simulink model "PMS_Motor_level4eZDSPF2812"  (Simulink 6.5)
settings: Solver=FixedStepDiscrete  StartTime=0.0  StopTime=0.3  RelTol=1e-3
libraries: simulink x13, tiiqmathlib x9, c28xdmclib x8, c281xdspchiplib x5, memblks x4, c2000tgtpreflib x1
CloseFcn:
  | rtwprivate ssgencode ModelCloseRequest Simple_DC_Motor
settings Model: Creator=JacobF  LastModifiedBy=JacobF  ProdHWDeviceType=TI C2000
settings DataIOCC: SaveOutput=off  SaveTime=off  SignalLoggingName=DataLog
settings OptimizationCC: OptimizeModelRefInitCode=on  LifeSpan=1
settings DebuggingCC: ReadBeforeWriteMsg=DisableAll  MultiTaskDSMMsg=warning  MultiTaskCondExecSysMsg=none  ParameterPrecisionLossMsg=none  StrictBusMsg=ErrorLevel1
settings HardwareCC: ProdBitPerChar=16  ProdBitPerInt=16  ProdIntDivRoundTo=Zero  ProdEndianess=LittleEndian  ProdWordSize=16  ProdHWDeviceType=TI C2000  TargetHWDeviceType=32-bit Generic
settings RTWCC: SystemTargetFile=ti_c2000_ert.tlc  GenCodeOnly=on  TemplateMakefile=ti_c2000_ert.tmf  Description=Embedded Target for TI C2000 DSP (ERT)  GenerateReport=on  ProcessScript=ti_c2000_ert_make_rtw_hook  IncludeHyperlinkInReport=on  LaunchReport=on
settings CodeAppCC: IgnoreCustomStorageClasses=off
settings STFCustomTargetCC: TargetFcnLib=ansi_tfl_tmw.mat  GenFloatMathFcnCalls=ANSI_C  ModelReferenceCompliant=off  CombineOutputUpdateFcns=on  ERTCustomFileBanners=on  SystemTargetFile=ti_c2000_ert.tlc
settings ERTTargetCC: TargetFcnLib=ansi_tfl_tmw.mat  GenFloatMathFcnCalls=ANSI_C  ModelReferenceCompliant=off  SupportContinuousTime=on  SupportNonInlinedSFcns=on  InlinedParameterPlacement=NonHierarchical  ERTCustomFileTemplate=example_file_process.tlc

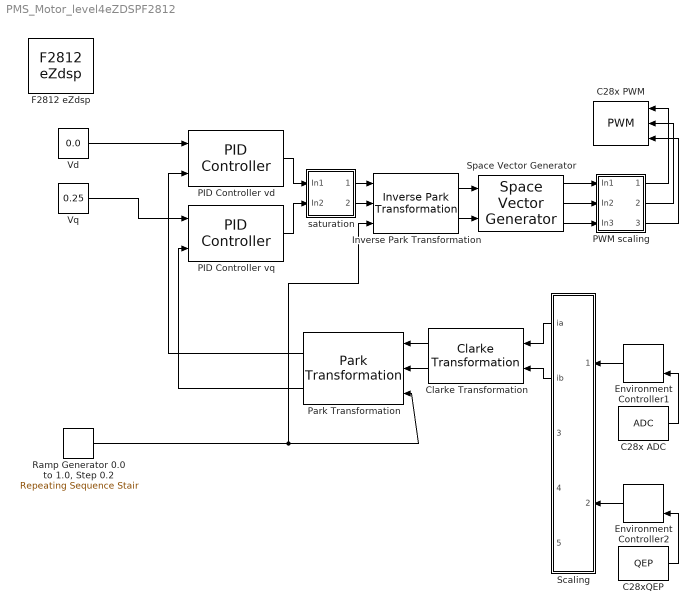
== system PMS_Motor_level4eZDSPF2812 ==
  C28x ADC : c281xdspchiplib/ADC  useModule=A  useMode=Sequential  sourceSOC=Software  Ts=-1  dType=uint16  postInterrupt=off  numConversionsSingle=3  numConversionsDouble=1  conv0=ADCINB0  conv1=ADCINB1  conv2=ADCINB2  conv3=ADCINB3  conv4=ADCINA4  conv5=ADCINA5  conv6=ADCINB6  conv7=ADCINA7  conv8=ADCINB0  conv9=ADCINB1  conv10=ADCINB2  conv11=ADCINB3  conv12=ADCINB4  conv13=ADCINB5  conv14=ADCINB6  conv15=ADCINB7  convAB0=ADCINA0 and ADCINB0  convAB1=ADCINA1 and ADCINB1  convAB2=ADCINA5 and ADCINB5  convAB3=ADCINA1 and ADCINB1  convAB4=ADCINA1 and ADCINB1  convAB5=ADCINA1 and ADCINB1  convAB6=ADCINA1 and ADCINB1  convAB7=ADCINA1 and ADCINB1  convA0=ADCINA0  convA1=ADCINA1  convA2=ADCINA7  convA3=ADCINA3  convA4=ADCINA4  convA5=ADCINA5  convA6=ADCINA6  convA7=ADCINA7  convB0=ADCINB0  convB1=ADCINB1  convB2=ADCINB2  convB3=ADCINB3  convB4=ADCINB4  convB5=ADCINB5  convB6=ADCINB6  convB7=ADCINB7  c28xmultiPort=off
  C28x PWM : c281xdspchiplib/PWM  Orientation=left  useModule=A  timerSource=Specify via dialog  timerPeriod=(2^12)+1  waveformType=Symmetric  periodUnits=Clock cycles  unit1Status=on  unit1Source=Input port  unit1Value=4096  unit2Status=on  unit2Source=Input port  unit2Value=4096  unit3Status=on  unit3Source=Input port  unit3Value=4096  dutyCycleUnits=Clock cycles  logicSource=Specify via dialog  unit1_1Logic=Active high  unit1_2Logic=Active low  unit2_1Logic=Active high  unit2_2Logic=Active low  unit3_1Logic=Active high  unit3_2Logic=Active low  enableDeadband1=on  enableDeadband2=on  enableDeadband3=on  deadbandPrescaler=8  deadbandPeriodSource=Specify via dialog  deadbandPeriod=15  adcstartEvent=None
  C28xQEP : c281xdspchiplib/QEP  useModule=A  countingMode=Counter  positiveRotation=Clockwise  initialCount=0  encoderResolution=1024  sampleTime=5e-5  dataType=uint16
  Clarke Transformation : c28xdmclib/Clarke Transformation  Orientation=left
  Environment Controller1 : simulink/Signal Routing/Environment Controller  Orientation=left  SystemSampleTime=-1
  Environment Controller2 : simulink/Signal Routing/Environment Controller  Orientation=left  SystemSampleTime=-1
  F2812 eZdsp : c2000tgtpreflib/F2812 eZdsp  Tag=C2000 TARGET PREFERENCES BLOCK  SystemSampleTime=-1
  Inverse Park Transformation : c28xdmclib/Inverse Park Transformation
  PID Controller vd : c28xdmclib/PID Controller  proportionalGain=0.2  integralGain=0.002  correctionGain=0.002  derivativeGain=0  minOutput=-1  maxOutput=1
  PID Controller vq : c28xdmclib/PID Controller  proportionalGain=0.2  integralGain=0.002  correctionGain=0.002  derivativeGain=0  minOutput=-1  maxOutput=1
  PWM scaling : Subsystem
  Park Transformation : c28xdmclib/Park Transformation  Orientation=left
  "Ramp Generator 0.0 to 1.0, Step 0.2" : simulink/Sources/Repeating Sequence Stair  SystemSampleTime=-1  OutValues=[0.0:0.0005:1.0]  tsamp=0.00005  OutputDataTypeScalingMode=Specify via dialog  OutDataType=sfix(32)  ConRadixGroup=Use Specified Scaling  OutScaling=2^-17
  Scaling : Subsystem  Orientation=left
  Space Vector Generator : c28xdmclib/Space Vector Generator
  Vd : Constant  Value=0.0  OutDataTypeMode=Specify via dialog  OutDataType=sfix(32)  ConRadixGroup=Use specified scaling  OutScaling=2^-17  SampleTime=inf  FramePeriod=inf
  Vq : Constant  Value=0.25  OutDataTypeMode=Specify via dialog  OutDataType=sfix(32)  ConRadixGroup=Use specified scaling  OutScaling=2^-17  SampleTime=inf  FramePeriod=inf
  saturation : Subsystem
  wires:
  Inverse Park Transformation/1 -> Space Vector Generator/1
  Inverse Park Transformation/2 -> Space Vector Generator/2
  Space Vector Generator/1 -> PWM scaling/1(In1)
  Space Vector Generator/2 -> PWM scaling/2(In2)
  Space Vector Generator/3 -> PWM scaling/3(In3)
  PWM scaling/1(Out1) -> C28x PWM/1
  PWM scaling/2(Out2) -> C28x PWM/2
  PWM scaling/3(Out3) -> C28x PWM/3
  C28xQEP/1 -> Environment Controller2/2
  Environment Controller1/1 -> Scaling/1(ADC)
  C28x ADC/1 -> Environment Controller1/2
  Environment Controller2/1 -> Scaling/2(QEP)
  Scaling/1(ia) -> Clarke Transformation/1
  Scaling/2(ib) -> Clarke Transformation/2
  Clarke Transformation/1 -> Park Transformation/1
  Clarke Transformation/2 -> Park Transformation/2
  PID Controller vd/1 -> saturation/1(In1)
  PID Controller vq/1 -> saturation/2(In2)
  Vd/1 -> PID Controller vd/1
  Park Transformation/1 -> PID Controller vd/2
  Park Transformation/2 -> PID Controller vq/2
  saturation/1(Out1) -> Inverse Park Transformation/1
  saturation/2(Out2) -> Inverse Park Transformation/2
  Vq/1 -> PID Controller vq/1
  "Ramp Generator 0.0 to 1.0, Step 0.2"/1 -> Inverse Park Transformation/3, Park Transformation/3

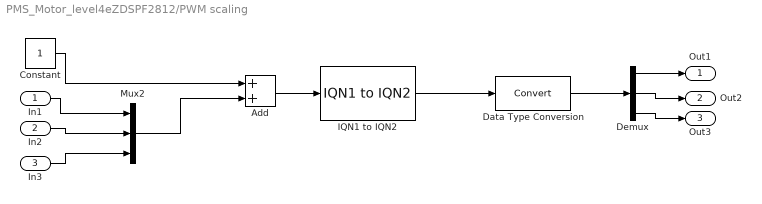
== system PMS_Motor_level4eZDSPF2812/PWM scaling ==
  In1 : Inport
  In2 : Inport  Port=2
  In3 : Inport  Port=3
  Add : Sum  OutScaling=2^-10
  Constant : Constant  Value=1  OutDataTypeMode=Specify via dialog  OutDataType=sfix(32)  ConRadixGroup=Use specified scaling  OutScaling=2^-17  SampleTime=inf  FramePeriod=inf
  Data Type Conversion : DataTypeConversion  OutDataTypeMode=uint16  ConvertRealWorld=Stored Integer (SI)
  Demux : Demux  Outputs=3
  IQN1 to IQN2 : tiiqmathlib/IQN1 to IQN2  New_Q=11
  Mux2 : Mux  Inputs=3
  Out1 : Outport
  Out2 : Outport  Port=2
  Out3 : Outport  Port=3
  wires:
  In1/1 -> Mux2/1
  Add/1 -> IQN1 to IQN2/1
  Constant/1 -> Add/1
  IQN1 to IQN2/1 -> Data Type Conversion/1
  In3/1 -> Mux2/3
  In2/1 -> Mux2/2
  Mux2/1 -> Add/2
  Data Type Conversion/1 -> Demux/1
  Demux/3 -> Out3/1
  Demux/2 -> Out2/1
  Demux/1 -> Out1/1

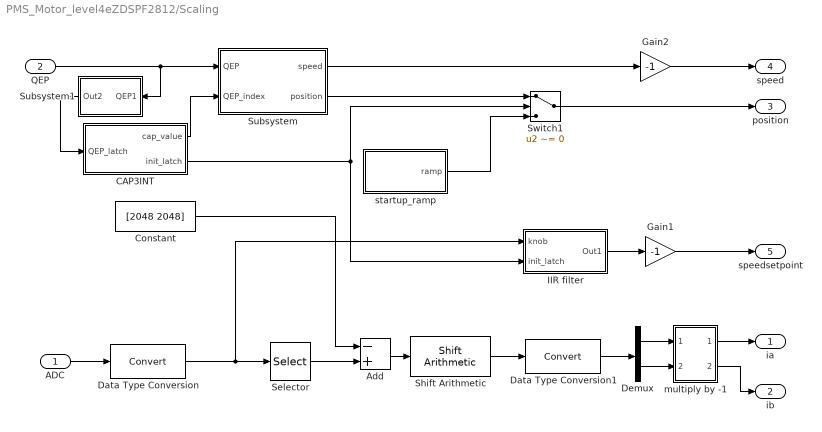
== system PMS_Motor_level4eZDSPF2812/Scaling ==
  ADC : Inport
  QEP : Inport  Port=2
  Add : Sum  Inputs=-+  OutScaling=2^-10
  CAP3INT : Subsystem
  Constant : Constant  Value=[2048 2048]  OutDataTypeMode=int32  OutDataType=sfix(32)  ConRadixGroup=Use specified scaling  OutScaling=2^-12  SampleTime=inf  FramePeriod=inf
  Data Type Conversion : DataTypeConversion  OutDataTypeMode=int32  OutDataType=sfix(32)  OutScaling=2^-12  ConvertRealWorld=Stored Integer (SI)
  Data Type Conversion1 : DataTypeConversion  OutDataTypeMode=Specify via dialog  OutDataType=sfix(32)  OutScaling=2^-17  ConvertRealWorld=Stored Integer (SI)
  Demux : Demux  Outputs=2
  Gain1 : Gain  Gain=-1
  Gain2 : Gain  Gain=-1
  IIR filter : Subsystem
  Selector : Selector  InputType=Vector  ElementSrc=Internal  Elements=[1 2]  RowSrc=Internal  Rows=1  ColumnSrc=Internal  Columns=1  InputPortWidth=3  IndexIsStartValue=off
  Shift Arithmetic : simulink/Logic and Bit Operations/Shift Arithmetic  SystemSampleTime=-1  nBitShiftRight=-6  nBinPtShiftRight=0
  Subsystem : Subsystem
  Subsystem1 : Subsystem  Orientation=left
      settings: RTWMemSecFuncInitTerm=Default  RTWMemSecFuncExecute=Default  RTWMemSecDataConstants=Default  RTWMemSecDataInternal=Default  RTWMemSecDataParameters=Default
  Switch1 : Switch  Criteria=u2 ~= 0
  multiply by -1 : Subsystem
  startup_ramp : Subsystem
  ia : Outport
  ib : Outport  Port=2
  position : Outport  Port=3
  speed : Outport  Port=4
  speedsetpoint : Outport  Port=5
  wires:
  Subsystem1/1(Out2) -> CAP3INT/1(QEP_latch)
  Switch1/1 -> position/1
  ADC/1 -> Data Type Conversion/1
  QEP/1 -> Subsystem/1(QEP), Subsystem1/1(QEP1)
  multiply by -1/2(Out2) -> ib/1
  multiply by -1/1(Out1) -> ia/1
  Demux/2 -> multiply by -1/2(In2)
  Demux/1 -> multiply by -1/1(In1)
  Data Type Conversion1/1 -> Demux/1
  Shift Arithmetic/1 -> Data Type Conversion1/1
  Add/1 -> Shift Arithmetic/1
  Selector/1 -> Add/2
  Constant/1 -> Add/1
  IIR filter/1(Out1) -> Gain1/1
  Data Type Conversion/1 -> IIR filter/1(knob), Selector/1
  Subsystem/2(position) -> Switch1/1
  Subsystem/1(speed) -> Gain2/1
  startup_ramp/1(ramp) -> Switch1/3
  CAP3INT/2(init_latch) -> IIR filter/2(init_latch), Switch1/2
  CAP3INT/1(cap_value) -> Subsystem/2(QEP_index)
  Gain2/1 -> speed/1
  Gain1/1 -> speedsetpoint/1

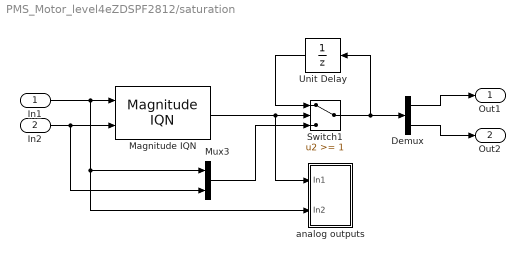
== system PMS_Motor_level4eZDSPF2812/saturation ==
  In1 : Inport
  In2 : Inport  Port=2
  Demux : Demux  Outputs=2
  Magnitude IQN : tiiqmathlib/Magnitude IQN
  Mux3 : Mux  Inputs=2
  Switch1 : Switch  Threshold=1
  Unit Delay : UnitDelay  Orientation=left  X0=[0 0]  SampleTime=-1
  analog outputs : Subsystem
  Out1 : Outport
  Out2 : Outport  Port=2
  wires:
  Magnitude IQN/1 -> Switch1/2, analog outputs/1(In1)
  In1/1 -> Magnitude IQN/1, Mux3/1, analog outputs/2(In2)
  In2/1 -> Magnitude IQN/2, Mux3/2
  Mux3/1 -> Switch1/3
  Switch1/1 -> Unit Delay/1, Demux/1
  Unit Delay/1 -> Switch1/1
  Demux/1 -> Out1/1
  Demux/2 -> Out2/1

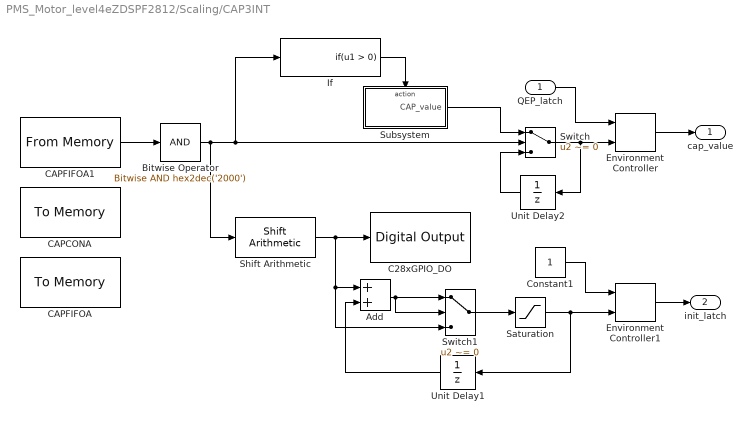
== system PMS_Motor_level4eZDSPF2812/Scaling/CAP3INT ==
  QEP_latch : Inport
  Add : Sum  OutDataTypeMode=uint16  OutScaling=2^-10
  Bitwise Operator : simulink/Logic and Bit Operations/Bitwise Operator  logicop=AND  UseBitMask=on  BitMask=hex2dec('2000')  BitMaskRealWorld=Stored Integer
  C28xGPIO_DO : c281xdspchiplib/Digital Output  useIOPort=GPIOB  GPIO_Bit0=off  GPIO_Bit1=off  GPIO_Bit2=off  GPIO_Bit3=off  GPIO_Bit4=off  GPIO_Bit5=off  GPIO_Bit6=off  GPIO_Bit7=off  GPIO_Bit8=off  GPIO_Bit9=on  GPIO_Bit10=off  GPIO_Bit11=off  GPIO_Bit12=off  GPIO_Bit13=off  GPIO_Bit14=off  GPIO_Bit15=off
  CAPCONA : memblks/To Memory  memAddressMask=7420  dType=uint16  useInitValue=on  initValue=hex2dec('1004')  useTermValue=off  termValue=0  isRealtimeEnabled=off  emitCCBeforeWrite=off  emitCCAfterWrite=off
  CAPFIFOA : memblks/To Memory  memAddressMask=7422  dType=uint16  useInitValue=on  initValue=hex2dec('1000')  useTermValue=off  termValue=0  isRealtimeEnabled=off  emitCCBeforeWrite=off  emitCCAfterWrite=off
  CAPFIFOA1 : memblks/From Memory  memAddressMask=7422  dType=uint16  Ts=-1  frameSize=1
  Constant1 : Constant  Value=1  OutDataTypeMode=uint16  OutDataType=sfix(16)  ConRadixGroup=Use specified scaling  OutScaling=2^0  SampleTime=inf  FramePeriod=inf
  Environment Controller : simulink/Signal Routing/Environment Controller  SystemSampleTime=-1
  Environment Controller1 : simulink/Signal Routing/Environment Controller  SystemSampleTime=-1
  If : If  ShowElse=off
  Saturation : Saturate  UpperLimit=1  LowerLimit=0
  Shift Arithmetic : simulink/Logic and Bit Operations/Shift Arithmetic  SystemSampleTime=-1  nBitShiftRight=13  nBinPtShiftRight=0
  Subsystem : Subsystem  TreatAsAtomicUnit=on
  Switch : Switch  Criteria=u2 ~= 0
  Switch1 : Switch  Criteria=u2 ~= 0  InputSameDT=on
  Unit Delay1 : UnitDelay  Orientation=left  SampleTime=-1
  Unit Delay2 : UnitDelay  Orientation=left  SampleTime=-1
  cap_value : Outport
  init_latch : Outport  Port=2
  wires:
  Constant1/1 -> Environment Controller1/1
  Environment Controller1/1 -> init_latch/1
  QEP_latch/1 -> Environment Controller/1
  Environment Controller/1 -> cap_value/1
  Saturation/1 -> Environment Controller1/2, Unit Delay1/1
  Switch1/1 -> Saturation/1
  Add/1 -> Switch1/1, Switch1/2
  Unit Delay1/1 -> Add/2
  Shift Arithmetic/1 -> Switch1/3, Add/1, C28xGPIO_DO/1
  Bitwise Operator/1 -> Shift Arithmetic/1, Switch/2, If/1
  If/1 -> Subsystem/Action
  Unit Delay2/1 -> Switch/3
  Switch/1 -> Environment Controller/2, Unit Delay2/1
  Subsystem/1(CAP_value) -> Switch/1
  CAPFIFOA1/1 -> Bitwise Operator/1

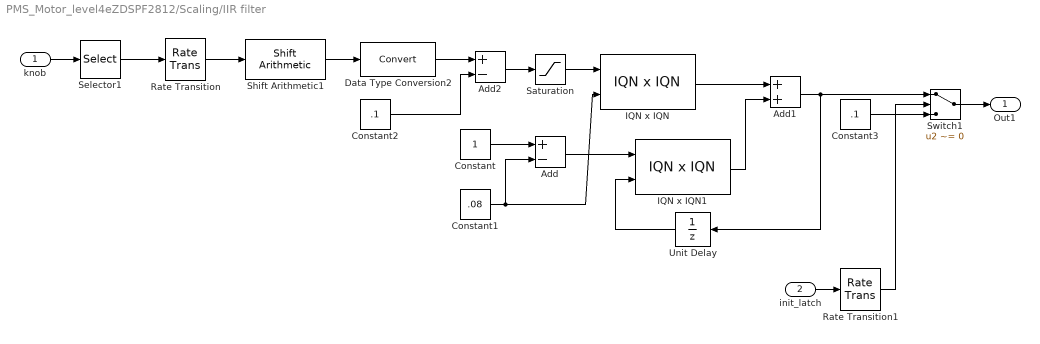
== system PMS_Motor_level4eZDSPF2812/Scaling/IIR filter ==
  knob : Inport
  init_latch : Inport  Port=2
  Add : Sum  Inputs=+-  OutScaling=2^-10
  Add1 : Sum  OutScaling=2^-10
  Add2 : Sum  Inputs=+-  OutScaling=2^-10
  Constant : Constant  Value=1  OutDataTypeMode=Specify via dialog  OutDataType=sfix(32)  ConRadixGroup=Use specified scaling  OutScaling=2^-17  SampleTime=inf  FramePeriod=inf
  Constant1 : Constant  Value=.08  OutDataTypeMode=Specify via dialog  OutDataType=sfix(32)  ConRadixGroup=Use specified scaling  OutScaling=2^-17  SampleTime=inf  FramePeriod=inf
  Constant2 : Constant  Value=.1  OutDataTypeMode=Specify via dialog  OutDataType=sfix(32)  ConRadixGroup=Use specified scaling  OutScaling=2^-17  SampleTime=inf  FramePeriod=inf
  Constant3 : Constant  Value=.1  OutDataTypeMode=Specify via dialog  OutDataType=sfix(32)  ConRadixGroup=Use specified scaling  OutScaling=2^-17  SampleTime=inf  FramePeriod=inf
  Data Type Conversion2 : DataTypeConversion  OutDataTypeMode=Specify via dialog  OutDataType=sfix(32)  OutScaling=2^-17  ConvertRealWorld=Stored Integer (SI)
  IQN x IQN : tiiqmathlib/IQN x IQN  multiplyOption=Multiply
  IQN x IQN1 : tiiqmathlib/IQN x IQN  multiplyOption=Multiply
  Rate Transition : RateTransition  Integrity=off  OutPortSampleTime=0.01
  Rate Transition1 : RateTransition  Integrity=off  OutPortSampleTime=0.01
  Saturation : Saturate  UpperLimit=1  LowerLimit=0
  Selector1 : Selector  InputType=Vector  ElementSrc=Internal  Elements=[3]  RowSrc=Internal  Rows=1  ColumnSrc=Internal  Columns=1  InputPortWidth=3  IndexIsStartValue=off
  Shift Arithmetic1 : simulink/Logic and Bit Operations/Shift Arithmetic  SystemSampleTime=-1  nBitShiftRight=-5  nBinPtShiftRight=0
  Switch1 : Switch  Criteria=u2 ~= 0
  Unit Delay : UnitDelay  Orientation=left  SampleTime=-1
  Out1 : Outport
  wires:
  Saturation/1 -> IQN x IQN/1
  Rate Transition/1 -> Shift Arithmetic1/1
  Rate Transition1/1 -> Switch1/2
  Switch1/1 -> Out1/1
  Constant3/1 -> Switch1/3
  init_latch/1 -> Rate Transition1/1
  Add2/1 -> Saturation/1
  Data Type Conversion2/1 -> Add2/1
  Constant2/1 -> Add2/2
  Shift Arithmetic1/1 -> Data Type Conversion2/1
  IQN x IQN1/1 -> Add1/2
  Unit Delay/1 -> IQN x IQN1/2
  Add1/1 -> Switch1/1, Unit Delay/1
  Add/1 -> IQN x IQN1/1
  IQN x IQN/1 -> Add1/1
  Constant1/1 -> IQN x IQN/2, Add/2
  Constant/1 -> Add/1
  knob/1 -> Selector1/1
  Selector1/1 -> Rate Transition/1

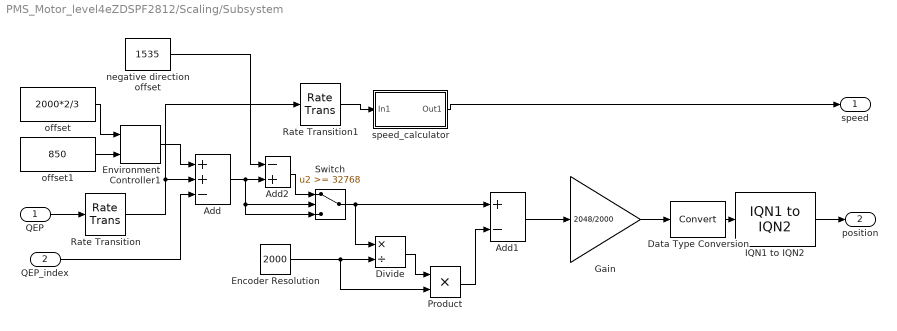
== system PMS_Motor_level4eZDSPF2812/Scaling/Subsystem ==
  QEP : Inport
  QEP_index : Inport  Port=2
  Add : Sum  Inputs=++-  OutScaling=2^-10
  Add1 : Sum  Inputs=+-  OutDataTypeMode=uint16  OutScaling=2^-10  RndMeth=Nearest
  Add2 : Sum  Inputs=-+  OutScaling=2^-10
  Data Type Conversion : DataTypeConversion  OutDataTypeMode=Specify via dialog  OutDataType=sfix(32)  OutScaling=2^-11  ConvertRealWorld=Stored Integer (SI)
  Divide : Product  Inputs=*/  OutDataTypeMode=uint16  OutScaling=2^-10
  Encoder Resolution : Constant  Value=2000  OutDataTypeMode=uint16  OutDataType=sfix(16)  ConRadixGroup=Use specified scaling  OutScaling=2^0  SampleTime=inf  FramePeriod=inf
  Environment Controller1 : simulink/Signal Routing/Environment Controller  SystemSampleTime=-1
  Gain : Gain  Gain=2048/2000  ParameterDataTypeMode=Specify via dialog  ParameterDataType=float('single')
  IQN1 to IQN2 : tiiqmathlib/IQN1 to IQN2  New_Q=17
  Product : Product  OutDataTypeMode=uint16  RndMeth=Zero
  Rate Transition : RateTransition
  Rate Transition1 : RateTransition
  Switch : Switch  Threshold=32768
  negative direction offset : Constant  Value=1535  OutDataTypeMode=uint16  OutDataType=sfix(16)  ConRadixGroup=Use specified scaling  OutScaling=2^0  SampleTime=inf  FramePeriod=inf
  offset : Constant  Value=2000*2/3  OutDataTypeMode=uint16  OutDataType=sfix(16)  ConRadixGroup=Use specified scaling  OutScaling=2^0  SampleTime=inf  FramePeriod=inf
  offset1 : Constant  Value=850  OutDataTypeMode=uint16  OutDataType=sfix(16)  ConRadixGroup=Use specified scaling  OutScaling=2^0  SampleTime=inf  FramePeriod=inf
  speed_calculator : Subsystem
  speed : Outport
  position : Outport  Port=2
  wires:
  offset1/1 -> Environment Controller1/2
  Environment Controller1/1 -> Add/1
  offset/1 -> Environment Controller1/1
  Add1/1 -> Gain/1
  Rate Transition1/1 -> speed_calculator/1(In1)
  Rate Transition/1 -> Add/2, Rate Transition1/1
  QEP_index/1 -> Add/3
  QEP/1 -> Rate Transition/1
  speed_calculator/1(Out1) -> speed/1
  Switch/1 -> Add1/1, Divide/1
  Add2/1 -> Switch/1
  negative direction offset/1 -> Add2/1
  IQN1 to IQN2/1 -> position/1
  Data Type Conversion/1 -> IQN1 to IQN2/1
  Gain/1 -> Data Type Conversion/1
  Product/1 -> Add1/2
  Divide/1 -> Product/1
  Encoder Resolution/1 -> Divide/2, Product/2
  Add/1 -> Add2/2, Switch/2, Switch/3

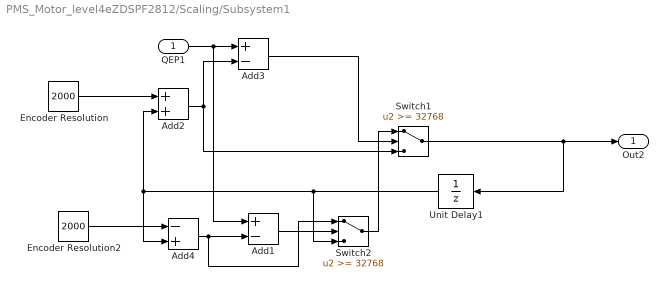
== system PMS_Motor_level4eZDSPF2812/Scaling/Subsystem1 ==
  QEP1 : Inport
  Add1 : Sum  Inputs=+-  OutDataTypeMode=uint16  OutScaling=2^-10
  Add2 : Sum  OutDataTypeMode=uint16  OutScaling=2^-10
  Add3 : Sum  Inputs=+-  OutDataTypeMode=uint16  OutScaling=2^-10
  Add4 : Sum  Inputs=-+  OutDataTypeMode=uint16  OutScaling=2^-10
  Encoder Resolution : Constant  Value=2000  OutDataTypeMode=uint16  OutDataType=sfix(16)  ConRadixGroup=Use specified scaling  OutScaling=2^0  SampleTime=inf  FramePeriod=inf
  Encoder Resolution2 : Constant  Value=2000  OutDataTypeMode=uint16  OutDataType=sfix(16)  ConRadixGroup=Use specified scaling  OutScaling=2^0  SampleTime=inf  FramePeriod=inf
  Switch1 : Switch  Threshold=32768
  Switch2 : Switch  Threshold=32768
  Unit Delay1 : UnitDelay  Orientation=left  SampleTime=-1
  Out2 : Outport
  wires:
  Encoder Resolution/1 -> Add2/1
  QEP1/1 -> Add3/1, Add1/1
  Add2/1 -> Add3/2, Switch1/3
  Add3/1 -> Switch1/2
  Switch1/1 -> Out2/1, Unit Delay1/1
  Unit Delay1/1 -> Add4/2, Add2/2, Switch2/3
  Encoder Resolution2/1 -> Add4/1
  Add4/1 -> Add1/2, Switch2/1
  Add1/1 -> Switch2/2
  Switch2/1 -> Switch1/1

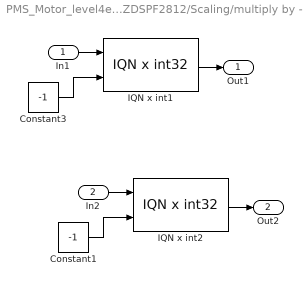
== system PMS_Motor_level4eZDSPF2812/Scaling/multiply by -1 ==
  In1 : Inport
  In2 : Inport  Port=2
  Constant1 : Constant  Value=-1  OutDataTypeMode=int32  OutDataType=sfix(32)  ConRadixGroup=Use specified scaling  OutScaling=2^-17  SampleTime=inf  FramePeriod=inf
  Constant3 : Constant  Value=-1  OutDataTypeMode=int32  OutDataType=sfix(32)  ConRadixGroup=Use specified scaling  OutScaling=2^-17  SampleTime=inf  FramePeriod=inf
  IQN x int1 : tiiqmathlib/IQN x int32
  IQN x int2 : tiiqmathlib/IQN x int32
  Out1 : Outport
  Out2 : Outport  Port=2
  wires:
  IQN x int2/1 -> Out2/1
  In2/1 -> IQN x int2/1
  Constant1/1 -> IQN x int2/2
  IQN x int1/1 -> Out1/1
  In1/1 -> IQN x int1/1
  Constant3/1 -> IQN x int1/2

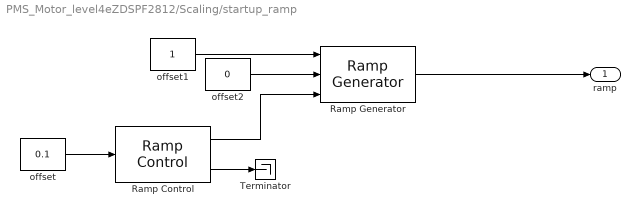
== system PMS_Motor_level4eZDSPF2812/Scaling/startup_ramp ==
  Ramp Control : c28xdmclib/Ramp Control  rmp_dly_max=1  rmp_lo_limit=0  rmp_hi_limit=1
  Ramp Generator : c28xdmclib/Ramp Generator  step_angle_max=0.005
  Terminator : Terminator
  offset : Constant  Value=0.1  OutDataTypeMode=Specify via dialog  OutDataType=sfix(32)  ConRadixGroup=Use specified scaling  OutScaling=2^-17  SampleTime=-1  FramePeriod=inf
  offset1 : Constant  Value=1  OutDataTypeMode=Specify via dialog  OutDataType=sfix(32)  ConRadixGroup=Use specified scaling  OutScaling=2^-17  SampleTime=-1  FramePeriod=inf
  offset2 : Constant  Value=0  OutDataTypeMode=Specify via dialog  OutDataType=sfix(32)  ConRadixGroup=Use specified scaling  OutScaling=2^-17  SampleTime=-1  FramePeriod=inf
  ramp : Outport
  wires:
  Ramp Generator/1 -> ramp/1
  offset1/1 -> Ramp Generator/1
  offset2/1 -> Ramp Generator/2
  Ramp Control/2 -> Terminator/1
  offset/1 -> Ramp Control/1
  Ramp Control/1 -> Ramp Generator/3

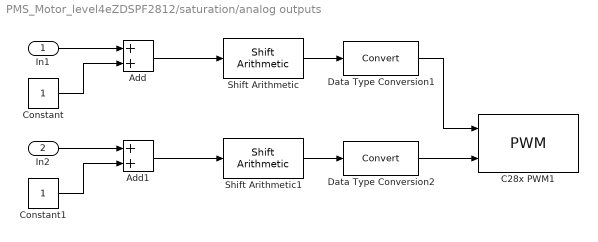
== system PMS_Motor_level4eZDSPF2812/saturation/analog outputs ==
  In1 : Inport
  In2 : Inport  Port=2
  Add : Sum  OutScaling=2^-10
  Add1 : Sum  OutScaling=2^-10
  C28x PWM1 : c281xdspchiplib/PWM  useModule=B  timerSource=Specify via dialog  timerPeriod=37500  waveformType=Symmetric  periodUnits=Clock cycles  unit1Status=on  unit1Source=Input port  unit1Value=18500  unit2Status=on  unit2Source=Input port  unit2Value=18500  unit3Status=off  unit3Source=Input port  unit3Value=18500  dutyCycleUnits=Clock cycles  logicSource=Specify via dialog  unit1_1Logic=Active high  unit1_2Logic=Active low  unit2_1Logic=Active high  unit2_2Logic=Active low  unit3_1Logic=Active high  unit3_2Logic=Active low  enableDeadband1=on  enableDeadband2=on  enableDeadband3=on  deadbandPrescaler=8  deadbandPeriodSource=Specify via dialog  deadbandPeriod=15  adcstartEvent=None
  Constant : Constant  Value=1  OutDataTypeMode=Specify via dialog  OutDataType=sfix(32)  ConRadixGroup=Use specified scaling  OutScaling=2^-17  SampleTime=inf  FramePeriod=inf
  Constant1 : Constant  Value=1  OutDataTypeMode=Specify via dialog  OutDataType=sfix(32)  ConRadixGroup=Use specified scaling  OutScaling=2^-17  SampleTime=inf  FramePeriod=inf
  Data Type Conversion1 : DataTypeConversion  OutDataTypeMode=uint16  OutDataType=sfix(32)  OutScaling=2^-17  ConvertRealWorld=Stored Integer (SI)
  Data Type Conversion2 : DataTypeConversion  OutDataTypeMode=uint16  OutDataType=sfix(32)  OutScaling=2^-17  ConvertRealWorld=Stored Integer (SI)
  Shift Arithmetic : simulink/Logic and Bit Operations/Shift Arithmetic  SystemSampleTime=-1  nBitShiftRight=3  nBinPtShiftRight=0
  Shift Arithmetic1 : simulink/Logic and Bit Operations/Shift Arithmetic  SystemSampleTime=-1  nBitShiftRight=3  nBinPtShiftRight=0
  wires:
  In1/1 -> Add/1
  Constant/1 -> Add/2
  Add/1 -> Shift Arithmetic/1
  Shift Arithmetic/1 -> Data Type Conversion1/1
  Data Type Conversion1/1 -> C28x PWM1/1
  In2/1 -> Add1/1
  Constant1/1 -> Add1/2
  Add1/1 -> Shift Arithmetic1/1
  Shift Arithmetic1/1 -> Data Type Conversion2/1
  Data Type Conversion2/1 -> C28x PWM1/2

== system PMS_Motor_level4eZDSPF2812/Scaling/CAP3INT/Subsystem ==
  Action Port : ActionPort  ActionType=then
  CAP1FBOT : memblks/From Memory  memAddressMask=7429  dType=uint16  Ts=-1  frameSize=1
  CAP_value : Outport
  wires:
  CAP1FBOT/1 -> CAP_value/1

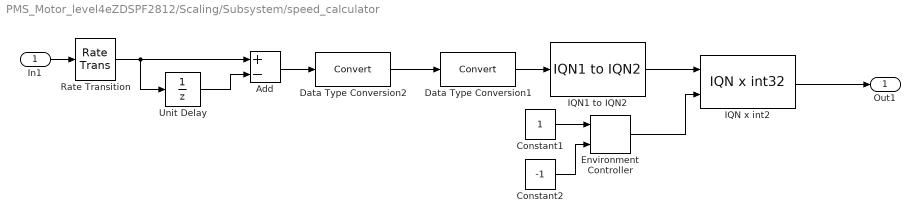
== system PMS_Motor_level4eZDSPF2812/Scaling/Subsystem/speed_calculator ==
  In1 : Inport
  Add : Sum  Inputs=+-  OutDataTypeMode=uint16  OutScaling=2^-10
  Constant1 : Constant  Value=1  OutDataTypeMode=int32  OutDataType=sfix(32)  ConRadixGroup=Use specified scaling  OutScaling=2^-17  SampleTime=inf  FramePeriod=inf
  Constant2 : Constant  Value=-1  OutDataTypeMode=int32  OutDataType=sfix(32)  ConRadixGroup=Use specified scaling  OutScaling=2^-17  SampleTime=inf  FramePeriod=inf
  Data Type Conversion1 : DataTypeConversion  OutDataTypeMode=Specify via dialog  OutDataType=sfix(32)  OutScaling=2^-10  ConvertRealWorld=Stored Integer (SI)
  Data Type Conversion2 : DataTypeConversion  OutDataTypeMode=int16  ConvertRealWorld=Stored Integer (SI)
  Environment Controller : simulink/Signal Routing/Environment Controller  SystemSampleTime=-1
  IQN x int2 : tiiqmathlib/IQN x int32
  IQN1 to IQN2 : tiiqmathlib/IQN1 to IQN2  New_Q=17
  Rate Transition : RateTransition  Integrity=off  OutPortSampleTime=0.01
  Unit Delay : UnitDelay  SampleTime=-1
  Out1 : Outport
  wires:
  Data Type Conversion2/1 -> Data Type Conversion1/1
  Data Type Conversion1/1 -> IQN1 to IQN2/1
  Add/1 -> Data Type Conversion2/1
  IQN1 to IQN2/1 -> IQN x int2/1
  Unit Delay/1 -> Add/2
  Rate Transition/1 -> Unit Delay/1, Add/1
  In1/1 -> Rate Transition/1
  IQN x int2/1 -> Out1/1
  Constant1/1 -> Environment Controller/1
  Constant2/1 -> Environment Controller/2
  Environment Controller/1 -> IQN x int2/2
